simulink model "servo_observer"  (R2019a)
settings: Solver=VariableStepAuto  StartTime=0.0  StopTime=18.0  RelTol=1e-3
values from neighbouring files (symbols this model uses):
  C = C(1:3,:)    [servo.m]
  K = real(inv(R)*Bbar'*P)    [servo.m]
  L = K_'    [servo.m]
undefined symbols (not defined in the file or in its folder): A, B, x0, ysp
settings Model: Creator=0210s  LastModifiedBy=0210s

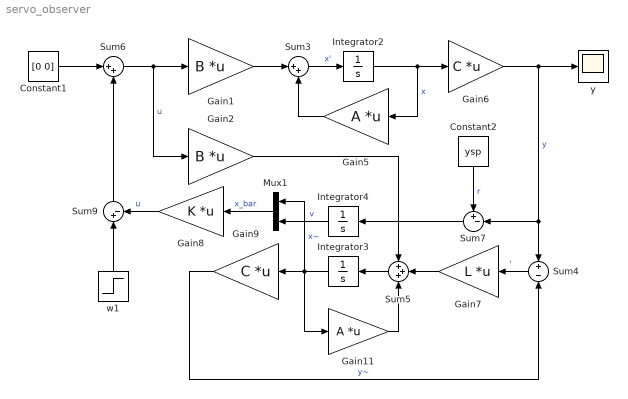
== system servo_observer ==
  Constant1 : Constant  Value=[0 0]
  Constant2 : Constant  Value=ysp
  Gain1 : Gain  Gain=B  Multiplication=Matrix(K*u) (u vector)
  Gain11 : Gain  Gain=A  Multiplication=Matrix(K*u) (u vector)
  Gain2 : Gain  Gain=B  Multiplication=Matrix(K*u) (u vector)
  Gain5 : Gain  Gain=A  Multiplication=Matrix(K*u) (u vector)
  Gain6 : Gain  Gain=C  Multiplication=Matrix(K*u) (u vector)
  Gain7 : Gain  Gain=L  Multiplication=Matrix(K*u) (u vector)
  Gain8 : Gain  Gain=K  Multiplication=Matrix(K*u) (u vector)
  Gain9 : Gain  Gain=C  Multiplication=Matrix(K*u) (u vector)
  Integrator2 : Integrator  InitialCondition=x0
  Integrator3 : Integrator  InitialCondition=[x0(1:3) 0 0 0]
  Integrator4 : Integrator
  Mux1 : Mux  Inputs=2
  Sum3 : Sum  Inputs=|++
  Sum4 : Sum  Inputs=+|-
  Sum5 : Sum  Inputs=+++
  Sum6 : Sum  Inputs=|++
  Sum7 : Sum  Inputs=+-|
  Sum9 : Sum  Inputs=|+-
  w1 : Step  Time=10  Before=[0 0]  After=[-1 1]  SampleTime=0  VectorParams1D=off
  y : Scope
  wires:
  Gain5/1 -> Sum3/2
  Gain1/1 -> Sum3/1
  Sum5/1 -> Integrator3/1
  Sum4/1 -> Gain7/1  "'"
  Sum3/1 -> Integrator2/1  "x'"
  Sum6/1 -> Gain2/1, Gain1/1  "u"
  Gain11/1 -> Sum5/3
  Integrator2/1 -> Gain5/1, Gain6/1  "x"
  Integrator3/1 -> Mux1/1, Gain11/1, Gain9/1  "x~"
  Constant1/1 -> Sum6/1
  Gain9/1 -> Sum4/2  "y~"
  Gain7/1 -> Sum5/2
  Constant2/1 -> Sum7/1  "r"
  Sum7/1 -> Integrator4/1
  Integrator4/1 -> Mux1/2  "v"
  w1/1 -> Sum9/1
  Gain8/1 -> Sum9/2  "u"
  Sum9/1 -> Sum6/2
  Mux1/1 -> Gain8/1  "x_bar"
  Gain6/1 -> y/1, Sum4/1, Sum7/2  "y"
  Gain2/1 -> Sum5/1
